simulink model "diagramablocos"  (R2015a)
settings: Solver=ode45  StartTime=0.0  StopTime=50.0  RelTol=1e-3
values from neighbouring files (symbols this model uses):
  tau = tauu(i)    [primeirolab.m]
  v0 = -3    [primeirolab.m]
  y = -0.55    [primeirolab.m]
settings Model: Creator=abran  LastModifiedBy=Pedro

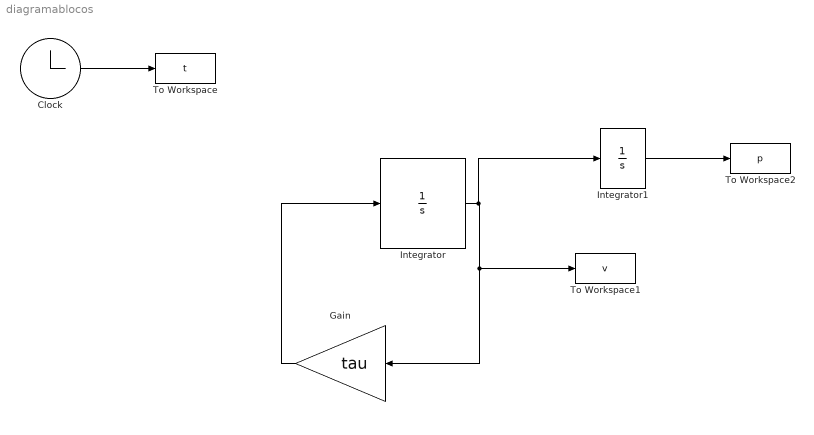
== system diagramablocos ==
  Clock : Clock
  Gain : Gain  Gain=tau
  Integrator : Integrator  InitialCondition=v0
  Integrator1 : Integrator  InitialCondition=y
  To Workspace : ToWorkspace  VariableName=t  SampleTime=-1
      settings: MaxDataPoints=1000000
  To Workspace1 : ToWorkspace  VariableName=v  SampleTime=-1
      settings: Save2DSignal=2-D array (concatenate along first dimension)
  To Workspace2 : ToWorkspace  VariableName=p  SampleTime=-1
  wires:
  Clock/1 -> To Workspace/1
  Integrator/1 -> Integrator1/1, Gain/1, To Workspace1/1
  Gain/1 -> Integrator/1
  Integrator1/1 -> To Workspace2/1
